simulink model "comparePWM"  (R2023b)
settings: Solver=ode4  StartTime=0.0  StopTime=0.1  FixedStep=Ts  RelTol=1e-3
PreLoadFcn:
  | % Switching
  | fsw = 2e4;
  | Tsw = 1/fsw;
  | Ts = 1e-7;
  | N = 8; % Number of subcycles
  | 
  | DeadTime = 2*Ts; % minimum value
  | 
  | % Default Variants
  | Delay = DelayType.Delay;
  | Inverter = InverterType.Ideal;
  | PWM = PWMType.Def3PhasePWMGen;
  | PWMAccuracy = PWMAccuracyType.Sync;
  | Solver = SolverType.ode4;
  | 
  | % Load Variant Configurations
  | load FastPWMConfigurations.mat;
undefined symbols (not defined in the file or in its folder): TsPWM
libraries: simulink x19, eePwmGenerator x18, nesl_utility x9, ee_lib x7, eePwmGeneratorTwoLevel x3, fl_lib x2, eeGeneralControl x1, eeSinGeneratorThreePhase x1
settings Model: VariantConfigurationObject=FastPWM  Creator=promero  LastModifiedBy=gschrabe
settings SolverCC: ODENIntegrationMethod=ode1be
settings OptimizationCC: ReuseModelBlockBuffer=off
settings ModelReferenceCC: EnableRefExpFcnMdlSchedulingChecks=on

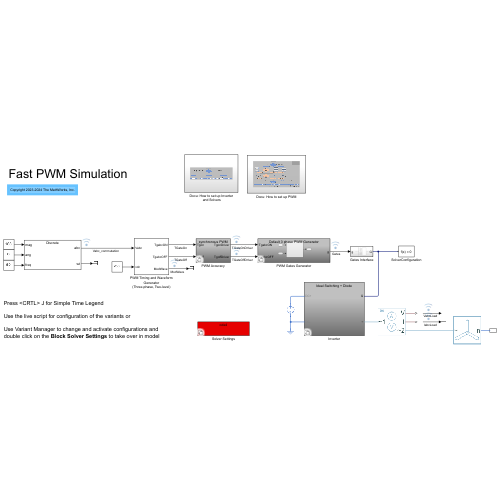
[thumbnail: Simulink's stored preview of the top-level diagram]
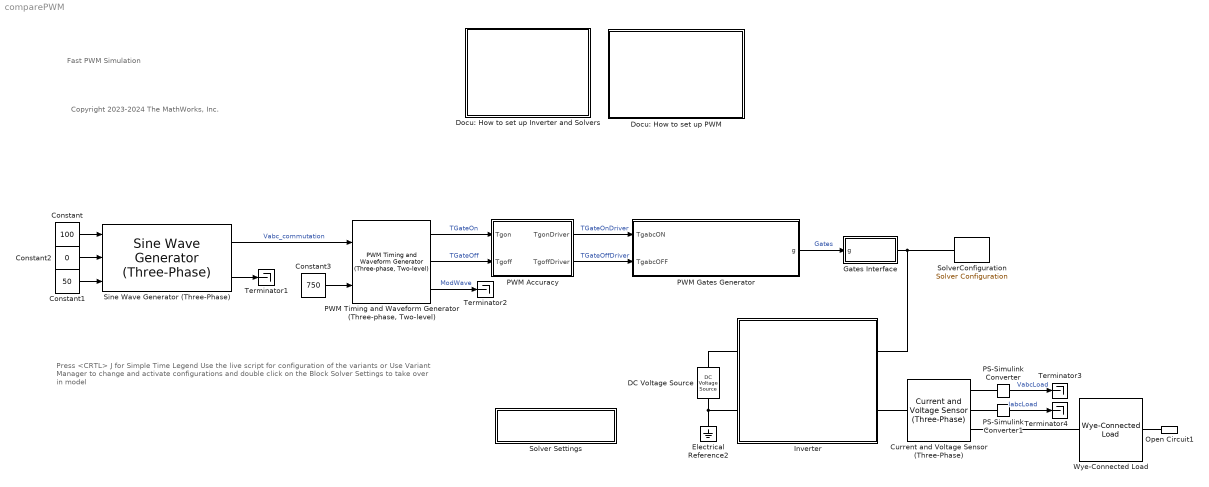
== system comparePWM ==
  note: Copyright 2023-2024 The MathWorks, Inc.
  note: Press <CRTL> J for Simple Time Legend
      |
      | Use the live script for configuration of the variants or
      |
      | Use Variant Manager to change and activate configurations and double click on the Block Solver Settings to take over in model
  note: Fast PWM Simulation
  Constant : Constant  Value=100  SampleTime=Tsw
  Constant1 : Constant  Value=50  SampleTime=Tsw
  Constant2 : Constant  Value=0  SampleTime=Tsw
  Constant3 : Constant  Value=750  SampleTime=Tsw
  Current and Voltage Sensor (Three-Phase) : ee_lib/Sensors & Transducers/Current and Voltage Sensor (Three-Phase)  vMeasurementType=ee.enum.vmeasurement.lg  outputUnit=ee.enum.unit.si  SRated=100e6 A*V  VRated=24e3 V  I_specify=off  I_priority=None  I=[0, 0, 0] A  I_nominal_specify=off  I_nominal_unit=A  I_nominal_value=1  V_specify=off  V_priority=None  V=[0, 0, 0] V  V_nominal_specify=off  V_nominal_unit=V  V_nominal_value=1
      settings: InternalSimscapePortConfiguration="{\"Bottom\":[],\"Left\":[{\"id\":\"N1\",\"label\":\"~1\",\"type\":\"foundation.electrical.three_phase\"}],\"Right\":[{\"id\":\"V_output\",\"label\":\"V\",\"type\":\"output\"},{\"id\":\"I_output\",\"label\":\"I\",\"type\":\"output\"},{\"id\":\"N2\",\"label\":\"~2\",\"type\":\"foundation.electrical.three_phase\"}],\"Top\":[]}"
  DC Voltage Source : ee_lib/Additional Components/SPICE Sources/DC Voltage Source  DC=750 V
  Docu: How to set up Inverter and Solvers : Subsystem
  Docu: How to set up PWM : Subsystem
  Electrical Reference2 : fl_lib/Electrical/Electrical Elements/Electrical Reference
  Gates Interface : Subsystem
  Inverter : Subsystem  Variant=on  VariantControl=Choice
  Open Circuit1 : fl_lib/Electrical/Electrical Elements/Open Circuit  v_specify=off  v_priority=None  v=0 V  v_nominal_specify=off  v_nominal_unit=V  v_nominal_value=1
  PS-Simulink Converter : nesl_utility/PS-Simulink Converter  PhysicalDomain=network_engine_domain  SubClassName=ps_output  LeftPortType=input  RightPortType=output  PseudoPeriodic=off  Frequencies=[]  VectorFormat=inherit  Unit=inherit  AffineConversion=off
  PS-Simulink Converter1 : nesl_utility/PS-Simulink Converter  PhysicalDomain=network_engine_domain  SubClassName=ps_output  LeftPortType=input  RightPortType=output  PseudoPeriodic=off  Frequencies=[]  VectorFormat=inherit  Unit=inherit  AffineConversion=off
  PWM Accuracy : Subsystem  InitFcn=|  Variant=on  VariantControl=Choice
      | if Ts == 0
      |    PWMAccuracy = 0;% ContinuousPWM;
      | else
      |    PWMAccuracy = 1; %DiscretePWM;
      | end
  PWM Gates Generator : Subsystem  Variant=on  VariantControl=Choice
  "PWM Timing and Waveform Generator (Three-phase, Two-level)" : eePwmGeneratorTwoLevel/PWM Timing and Waveform Generator (Three-phase, Two-level)  PWMMode=Continuous PWM (CPWM)  CPWMMode=SVM: space vector modulation  DPWMMode=60 DPWM (-30 degree shift): -30 degree shift from 60 DPWM  fsw=fsw
      settings: SamplingMode=Symmetric
  Sine Wave Generator (Three-Phase) : eeSinGeneratorThreePhase/Sine Wave Generator (Three-Phase)  Ts=Tsw
  Solver Settings : Subsystem  Priority=1  Variant=on  VariantControl=Modelwide Solver Settings
      settings: OpenFcn=open_system(['comparePWM_modified/Solver Settings/',char(Solver)]);
  SolverConfiguration : nesl_utility/Solver Configuration  PhysicalDomain=network_engine_domain  SubClassName=solver  LeftPortType=input  RightPortType=generic  Tones=[]  Harmonics=[]  SimulateNoise=off  Profile=off  UseLocalSampling=off  EnableSwitchedLinearOptims=on  FrequencyDomain=off  UseCCode=off  RelTol=0.001  AbsTol=0.001  MinStep=1e-09  ToWorkspace=off  RevertToSquareIcSolve=off  NumHomotopyIterations=100  PhasorMode=off  PhasorModeNumHarmonics=1  ConsistencySolver=NEWTON_FTOL  IndexReductionMethod=DerivativeReplacement  DoDC=off  ResidualTolerance=1e-09  ConsistencyTolSource=GLOBAL  ConsistencyAbsTol=0.001  ConsistencyRelTol=0.001  ConsistencyTolFactor=0.001  UseLocalSolver=on  LocalSolverChoice=NE_BACKWARD_EULER_ADVANCER  ResolveIndetEquations=on  FunctionEvalNumThread=1  LocalSolverSampleTime=Ts  DoFixedCost=off  MaxNonlinIter=3  MaxModeIter=2  ComputeImpulses=off  ImpulseIterations=2  LinearAlgebra=auto  LinearAlgebraNumThread=0  EquationFormulation=NE_TIME_EF  DelaysMemoryBudget=1024  AutomaticFiltering=on  FilteringTimeConstant=0.001  PartitionStorageMethod=AS_NEEDED  PartitionMemoryBudget=1024  PartitionMethod=ROBUST  MultibodyUseLocalSolver=off  MultibodyLocalSolverChoice=ODE1  MultibodyLocalSolverSampleTime=0.001
  Terminator{1..4} (4 alike) : Terminator
  Wye-Connected Load : ee_lib/Passive/RLC Assemblies/Wye-Connected Load  parameterization=ee.enum.rlc.parameterization.direct  component_structure=ee.enum.rlc.structure.SeriesRL  component_structure_PQ=ee.enum.rlc.structure.SeriesRL  R=1 Ohm  L=1e-3 H  C=1e-6 F  VRated=24e3 V  FRated=60 Hz  P=1e3 W  Qpos=1e2 A*V  Qneg=-1e2 A*V  R_parasitic=0 Ohm  G_parasitic=0 1/Ohm  R_parasitic_PQ=0 Ohm  G_parasitic_PQ=0 1/Ohm  Vmag0=24e3 V  Vang0=0 deg  Freq0=60 Hz  IL_specify=off  IL_priority=High  IL=[0, 0, 0] A  IL_nominal_specify=off  IL_nominal_unit=A  IL_nominal_value=1  VC_specify=off  VC_priority=High  VC=[0, 0, 0] V  VC_nominal_specify=off  VC_nominal_unit=V  VC_nominal_value=1
  wires:
  Constant/1 -> Sine Wave Generator (Three-Phase)/1
  Constant1/1 -> Sine Wave Generator (Three-Phase)/3
  Sine Wave Generator (Three-Phase)/1 -> "PWM Timing and Waveform Generator (Three-phase, Two-level)"/1  "Vabc_commutation"
  Sine Wave Generator (Three-Phase)/2 -> Terminator1/1
  Constant2/1 -> Sine Wave Generator (Three-Phase)/2
  Constant3/1 -> "PWM Timing and Waveform Generator (Three-phase, Two-level)"/2
  "PWM Timing and Waveform Generator (Three-phase, Two-level)"/3 -> Terminator2/1  "ModWave"
  PS-Simulink Converter/1 -> Terminator3/1  "VabcLoad"
  PS-Simulink Converter1/1 -> Terminator4/1  "IabcLoad"
  PWM Gates Generator/1(g) -> Gates Interface/1(g)  "Gates"
  "PWM Timing and Waveform Generator (Three-phase, Two-level)"/1 -> PWM Accuracy/1(Tgon)  "TGateOn"
  "PWM Timing and Waveform Generator (Three-phase, Two-level)"/2 -> PWM Accuracy/2(Tgoff)  "TGateOff"
  PWM Accuracy/1(TgonDriver) -> PWM Gates Generator/1(TgabcON)  "TGateOnDriver"
  PWM Accuracy/2(TgoffDriver) -> PWM Gates Generator/2(TgabcOFF)  "TGateOffDriver"
  connections:
  Wye-Connected Load/LConn1 -- Current and Voltage Sensor (Three-Phase)/RConn3
  PS-Simulink Converter/LConn1 -- Current and Voltage Sensor (Three-Phase)/RConn1
  PS-Simulink Converter1/LConn1 -- Current and Voltage Sensor (Three-Phase)/RConn2
  DC Voltage Source/RConn1 -- Electrical Reference2/LConn1 -- Inverter/RConn2
  Inverter/LConn1 -- SolverConfiguration/RConn1 -- Gates Interface/RConn1
  Inverter/LConn2 -- Current and Voltage Sensor (Three-Phase)/LConn1
  Inverter/RConn1 -- DC Voltage Source/LConn1
  Wye-Connected Load/RConn1 -- Open Circuit1/LConn1

== system comparePWM/Docu: How to set up Inverter and Solvers ==

== system comparePWM/Docu: How to set up PWM ==

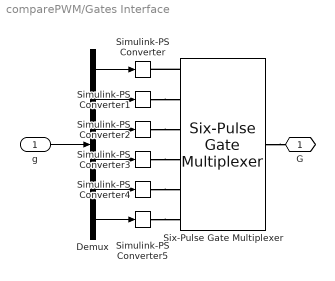
== system comparePWM/Gates Interface ==
  g : Inport
  Demux : Demux  Outputs=6
  Simulink-PS Converter{,1..5} (6 alike) : nesl_utility/Simulink-PS Converter  PhysicalDomain=network_engine_domain  SubClassName=ps_input  LeftPortType=input  RightPortType=output  PseudoPeriodic=off  Frequencies=[]  NoiseDistribution=none  NoiseParameters=[]  Unit=1  AffineConversion=off  FilteringAndDerivatives=provide  SimscapeFilterOrder=1  InputFilterTimeConstant=0.001  UdotUserProvided=0
  Six-Pulse Gate Multiplexer : ee_lib/Semiconductors & Converters/Converters/Six-Pulse Gate Multiplexer  port_option=ee.enum.controlport.ps
  G : PMIOPort  Side=Right
  wires:
  Demux/5 -> Simulink-PS Converter4/1
  Demux/1 -> Simulink-PS Converter/1
  Demux/4 -> Simulink-PS Converter3/1
  Demux/6 -> Simulink-PS Converter5/1
  Demux/2 -> Simulink-PS Converter1/1
  Demux/3 -> Simulink-PS Converter2/1
  g/1 -> Demux/1
  connections:
  Simulink-PS Converter5/RConn1 -- Six-Pulse Gate Multiplexer/LConn6
  Simulink-PS Converter1/RConn1 -- Six-Pulse Gate Multiplexer/LConn2
  Simulink-PS Converter4/RConn1 -- Six-Pulse Gate Multiplexer/LConn5
  Simulink-PS Converter2/RConn1 -- Six-Pulse Gate Multiplexer/LConn3
  Simulink-PS Converter3/RConn1 -- Six-Pulse Gate Multiplexer/LConn4
  Six-Pulse Gate Multiplexer/LConn1 -- Simulink-PS Converter/RConn1
  Six-Pulse Gate Multiplexer/RConn1 -- G/RConn1

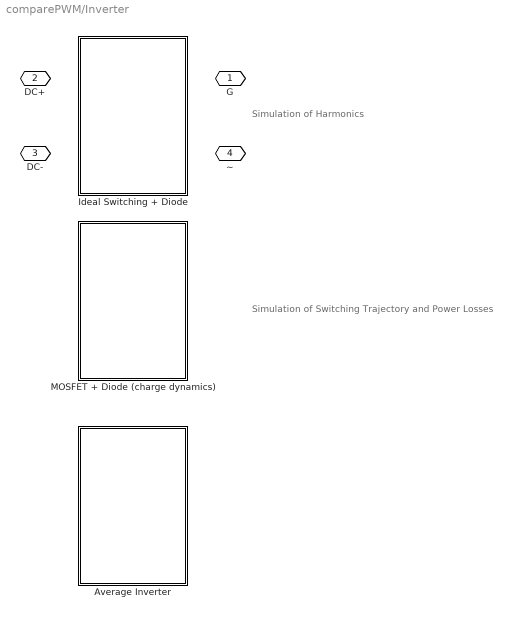
== system comparePWM/Inverter ==
  note: Simulation of Switching Trajectory and Power Losses
  note: Simulation of Harmonics
  Average Inverter : Subsystem  VariantControl=Inverter == InverterType.Average
  Ideal Switching + Diode : Subsystem  VariantControl=Inverter == InverterType.Ideal
  MOSFET + Diode (charge dynamics) : Subsystem  VariantControl=Inverter == InverterType.MOSFET
  G : PMIOPort  Side=Left
  DC+ : PMIOPort  Port=2  Side=Right
  DC- : PMIOPort  Port=3  Side=Right
  ~ : PMIOPort  Port=4  Side=Left

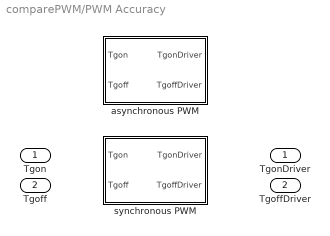
== system comparePWM/PWM Accuracy ==
  Tgon : Inport
  Tgoff : Inport  Port=2
  asynchronous PWM : Subsystem  VariantControl=PWMAccuracy == PWMAccuracyType.Async
  synchronous PWM : Subsystem  VariantControl=PWMAccuracy == PWMAccuracyType.Sync
  TgonDriver : Outport
  TgoffDriver : Outport  Port=2

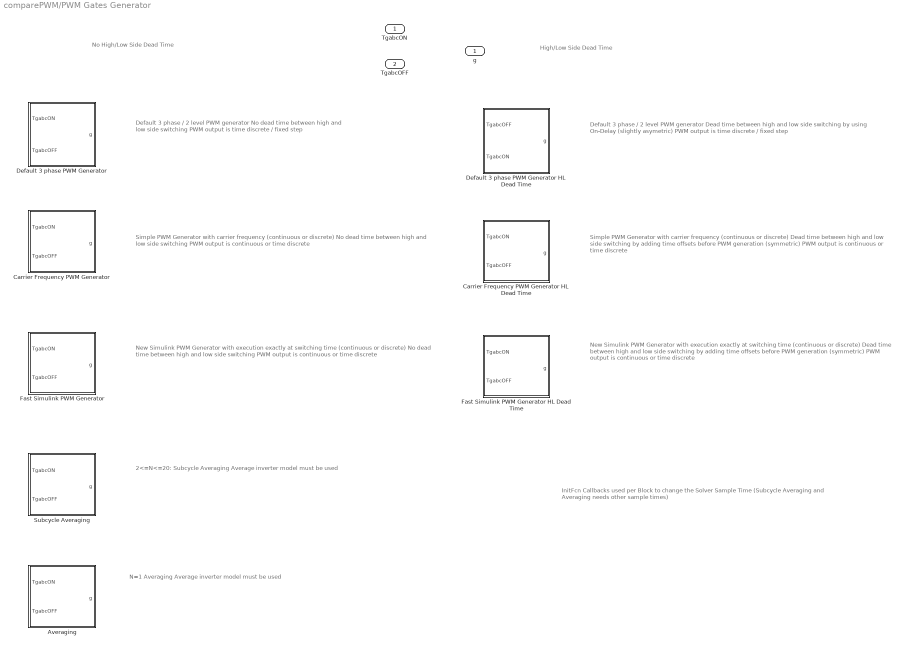
== system comparePWM/PWM Gates Generator ==
  note: InitFcn Callbacks used per Block to change the Solver Sample Time (Subcycle Averaging and Averaging needs other sample times)
  note: No High/Low Side Dead Time
  note: Default 3 phase / 2 level PWM generator
      | No dead time between high and low side switching
      | PWM output is time discrete / fixed step
  note: Default 3 phase / 2 level PWM generator
      | Dead time between high and low side switching by using On-Delay (slightly asymetric)
      | PWM output is time discrete / fixed step
  note: Simple PWM Generator with carrier frequency (continuous or discrete)
      | No dead time between high and low side switching
      | PWM output is continuous or time discrete
  note: Simple PWM Generator with carrier frequency (continuous or discrete)
      | Dead time between high and low side switching by adding time offsets before PWM generation (symmetric)
      | PWM output is continuous or time discrete
  note: New Simulink PWM Generator with execution exactly at switching time (continuous or discrete)
      | No dead time between high and low side switching
      | PWM output is continuous or time discrete
  note: New Simulink PWM Generator with execution exactly at switching time (continuous or discrete)
      | Dead time between high and low side switching by adding time offsets before PWM generation (symmetric)
      | PWM output is continuous or time discrete
  note: High/Low Side Dead Time
  note: 2<=N<=20: Subcycle Averaging
      | Average inverter model must be used
  note: N=1 Averaging
      | Average inverter model must be used
  TgabcON : Inport
  TgabcOFF : Inport  Port=2
  Averaging : Subsystem  InitFcn=|  VariantControl=PWM == PWMType.Averaging  mask{fsw=fsw, N=1}
      | set_param(bdroot,'FixedStep','Tsw');
      | set_param([bdroot,'/SolverConfiguration'],'LocalSolverSampleTime','Tsw');
      mask prompts: fsw "Switching frequency [Hz]"; N "Number of subcycles"
  Carrier Frequency PWM Generator : Subsystem  InitFcn=|  VariantControl=PWM == PWMType.CarrierFreqPWMGen  mask{fsw=fsw, Ts=TsPWM}
      | set_param(bdroot,'FixedStep','Ts');
      | set_param([bdroot,'/SolverConfiguration'],'LocalSolverSampleTime','Ts');
      mask prompts: fsw "Switching frequency [Hz]"; Ts "Sample Time"
  Carrier Frequency PWM Generator HL Dead Time : Subsystem  InitFcn=|  VariantControl=PWM == PWMType.CarrierFreqPWMGenHighLowDeadTime  mask{fsw=fsw, Ts=TsPWM, T_Dead=DeadTime}
      | set_param(bdroot,'FixedStep','Ts');
      | set_param([bdroot,'/SolverConfiguration'],'LocalSolverSampleTime','Ts');
      mask prompts: fsw "Switching frequency [Hz]"; Ts "Sample Time"; T_Dead "PWM dead time high/low side"
  Default 3 phase PWM Generator : Subsystem  InitFcn=|  VariantControl=PWM == PWMType.Def3PhasePWMGen
      | set_param(bdroot,'FixedStep','Ts');
      | set_param([bdroot,'/SolverConfiguration'],'LocalSolverSampleTime','Ts');
  Default 3 phase PWM Generator HL Dead Time : Subsystem  InitFcn=|  VariantControl=PWM == PWMType.Def3PhasePWMGenHighLowDeadTime  mask{fsw=fsw, Ts=Ts, T_Dead=DeadTime}
      | set_param(bdroot,'FixedStep','Ts');
      | set_param([bdroot,'/SolverConfiguration'],'LocalSolverSampleTime','Ts');
      mask prompts: fsw "Switching Frequency"; Ts "Sample Time"; T_Dead "PWM Dead Time High/Low side"
  Fast Simulink PWM Generator : Subsystem  ClipboardFcn=|  VariantControl=PWM == PWMType.FastSimulinkPWMGen  mask{fsw=fsw, Ts=TsPWM}
      | set_param(bdroot,'FixedStep','Ts');
      | set_param([bdroot,'/SolverConfiguration'],'LocalSolverSampleTime','Ts');
      mask prompts: fsw "Switching frequency [Hz]"; Ts "Sample Time"
      mask Callback Ts:
      | if evalin('base',get_param(gcb,'Ts')) == 0
      |         h = find_system(gcb,'LookUnderMasks','on','MatchFilter',@Simulink.match.allVariants,'RunAtFixedTimeIntervals','on');
      |         for i=1:length(h)
      |             set_param(h{i},'RunAtFixedTimeIntervals','off')
      |         end
      |     else
      |         h = find_system(gcb,'LookUnderMasks','on','MatchFilter',@Simulink.match.allVariants,'RunAtFixedTimeIntervals','off');
      |         for i=1:length(h)
      |             set_param(h{i},'RunAtFixedTimeIntervals','on')
      |         end
      |     end
  Fast Simulink PWM Generator HL Dead Time : Subsystem  InitFcn=|  VariantControl=PWM == PWMType.FastSimulinkPWMGenHighLowDeadTime  mask{fsw=fsw, T_Dead=DeadTime, Ts=TsPWM}
      | set_param(bdroot,'FixedStep','Ts');
      | set_param([bdroot,'/SolverConfiguration'],'LocalSolverSampleTime','Ts');
      mask prompts: fsw "Switching frequency [Hz]"; T_Dead "PWM dead time high/low side"; Ts "Sample Time"
      mask Callback Ts:
      | if evalin('base',get_param(gcb,'Ts')) == 0
      |         h = find_system(gcb,'LookUnderMasks','on','MatchFilter',@Simulink.match.allVariants,'RunAtFixedTimeIntervals','on');
      |         for i=1:length(h)
      |             set_param(h{i},'RunAtFixedTimeIntervals','off')
      |         end
      |     else
      |         h = find_system(gcb,'LookUnderMasks','on','MatchFilter',@Simulink.match.allVariants,'RunAtFixedTimeIntervals','off');
      |         for i=1:length(h)
      |             set_param(h{i},'RunAtFixedTimeIntervals','on')
      |         end
      |     end
  Subcycle Averaging : Subsystem  InitFcn=|  VariantControl=PWM == PWMType.SubcycleAvg  mask{fsw=fsw, N=N}
      | set_param(bdroot,'FixedStep','Tsw/N');
      | set_param([bdroot,'/SolverConfiguration'],'LocalSolverSampleTime','Tsw/N');
      mask prompts: fsw "Switching frequency [Hz]"; N "Number of subcycles"
  g : Outport

== system comparePWM/Solver Settings ==
  note: The global solver is changed depending on selected variant
      | This happens with predefined configuration sets
      | Also the Simscape lcoal solver setting is changed here.
  ode23t : Subsystem  VariantControl=Solver == SolverType.ode23t
      settings: OpenFcn=|
      | mdl = bdroot;
      | setActiveConfigSet(mdl,'ode23t');
      | set_param([mdl,'/SolverConfiguration'],'UseLocalSolver','off');
      | TsPWM = 0;
  ode4 : Subsystem  VariantControl=Solver == SolverType.ode4
      settings: OpenFcn=|
      | mdl = bdroot;
      | setActiveConfigSet(mdl,'ode4');
      | set_param([mdl,'/SolverConfiguration'],'UseLocalSolver','on');
      |         set_param([mdl,'/SolverConfiguration'],'LocalSolverChoice','NE_BACKWARD_EULER_ADVANCER');
      |         set_param([mdl,'/SolverConfiguration'],'LocalSolverSampleTime','Ts');
      | TsPWM = Ts;
  odeN : Subsystem  VariantControl=Solver == SolverType.odeN
      settings: OpenFcn=|
      | mdl = bdroot;
      | setActiveConfigSet(mdl,'odeN');
      | set_param([mdl,'/SolverConfiguration'],'UseLocalSolver','off');
      | TsPWM = 0;

== system comparePWM/Inverter/Average Inverter ==
  Converter (Three-Phase) : ee_lib/Semiconductors & Converters/Converters/Converter (Three-Phase)  port_option=ee.enum.threePhasePort.composite  device_type=ee.enum.converters.switchingdevice.averaged  K=0  Vf=0.8 V  Ron=0.001 Ohm  Rds=0.001 Ohm  Goff=1e-6 1/Ohm  Vgt=1 V  Vgt_off=-1 V  Ih=1 A  Vth=0.5 V  diode_param=ee.enum.converters.protectiondiode.chargedynamics  diode_Vf=0.8 V  diode_Ron=0.001 Ohm  diode_Goff=1e-5 1/Ohm  diode_C=50 nF  diode_iRM=-235 A  diode_iF=300 A  diode_idot=-50 A/us  diode_trr_param=ee.enum.converters.diodetrr.trr_factor  diode_trr_factor=3  diode_trr=15 us  diode_Qrr=1500 s*uA  snubber_type=ee.enum.converters.snubber.exclude  Cs=1e-7 F  Rs=0.1 Ohm
  G : PMIOPort  Side=Left
  DC+ : PMIOPort  Port=2  Side=Right
  DC- : PMIOPort  Port=3  Side=Right
  ~ : PMIOPort  Port=4  Side=Left
  connections:
  Converter (Three-Phase)/RConn1 -- DC+/RConn1
  Converter (Three-Phase)/RConn2 -- DC-/RConn1
  G/RConn1 -- Converter (Three-Phase)/LConn1
  ~/RConn1 -- Converter (Three-Phase)/LConn2

== system comparePWM/Inverter/Ideal Switching + Diode ==
  Converter (Three-Phase) : ee_lib/Semiconductors & Converters/Converters/Converter (Three-Phase)  port_option=ee.enum.threePhasePort.composite  device_type=ee.enum.converters.switchingdevice.ideal  K=0  Vf=0.8 V  Ron=0.001 Ohm  Rds=0.001 Ohm  Goff=1e-6 1/Ohm  Vgt=1 V  Vgt_off=-1 V  Ih=1 A  Vth=0.5 V  diode_param=ee.enum.converters.protectiondiode.nodynamics  diode_Vf=0.8 V  diode_Ron=0.001 Ohm  diode_Goff=1e-5 1/Ohm  diode_C=50 nF  diode_iRM=-235 A  diode_iF=300 A  diode_idot=-50 A/us  diode_trr_param=ee.enum.converters.diodetrr.trr_factor  diode_trr_factor=3  diode_trr=15 us  diode_Qrr=1500 s*uA  snubber_type=ee.enum.converters.snubber.exclude  Cs=1e-7 F  Rs=0.1 Ohm
  G : PMIOPort  Side=Left
  DC+ : PMIOPort  Port=2  Side=Right
  DC- : PMIOPort  Port=3  Side=Right
  ~ : PMIOPort  Port=4  Side=Left
  connections:
  Converter (Three-Phase)/RConn1 -- DC+/RConn1
  Converter (Three-Phase)/RConn2 -- DC-/RConn1
  G/RConn1 -- Converter (Three-Phase)/LConn1
  ~/RConn1 -- Converter (Three-Phase)/LConn2

== system comparePWM/Inverter/MOSFET + Diode (charge dynamics) ==
  Converter (Three-Phase) : ee_lib/Semiconductors & Converters/Converters/Converter (Three-Phase)  port_option=ee.enum.threePhasePort.composite  device_type=ee.enum.converters.switchingdevice.mosfet  K=0  Vf=0.8 V  Ron=0.001 Ohm  Rds=0.001 Ohm  Goff=1e-6 1/Ohm  Vgt=1 V  Vgt_off=-1 V  Ih=1 A  Vth=0.5 V  diode_param=ee.enum.converters.protectiondiode.chargedynamics  diode_Vf=0.8 V  diode_Ron=0.001 Ohm  diode_Goff=1e-5 1/Ohm  diode_C=50 nF  diode_iRM=-235 A  diode_iF=300 A  diode_idot=-50 A/us  diode_trr_param=ee.enum.converters.diodetrr.trr_factor  diode_trr_factor=3  diode_trr=15 us  diode_Qrr=1500 s*uA  snubber_type=ee.enum.converters.snubber.exclude  Cs=1e-7 F  Rs=0.1 Ohm
  G : PMIOPort  Side=Left
  DC+ : PMIOPort  Port=2  Side=Right
  DC- : PMIOPort  Port=3  Side=Right
  ~ : PMIOPort  Port=4  Side=Left
  connections:
  ~/RConn1 -- Converter (Three-Phase)/LConn2
  G/RConn1 -- Converter (Three-Phase)/LConn1
  Converter (Three-Phase)/RConn2 -- DC-/RConn1
  Converter (Three-Phase)/RConn1 -- DC+/RConn1

== system comparePWM/PWM Accuracy/asynchronous PWM ==
  note: Take exact PWM switching times
  Tgon : Inport
  Tgoff : Inport  Port=2
  TgonDriver : Outport
  TgoffDriver : Outport  Port=2
  wires:
  Tgoff/1 -> TgoffDriver/1
  Tgon/1 -> TgonDriver/1

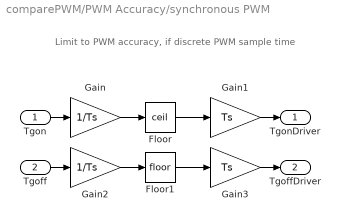
== system comparePWM/PWM Accuracy/synchronous PWM ==
  note: Limit to PWM accuracy, if discrete PWM sample time
  Tgon : Inport
  Tgoff : Inport  Port=2
  Floor : Rounding  Operator=ceil
  Floor1 : Rounding
  Gain : Gain  Gain=1/Ts
  Gain1 : Gain  Gain=Ts
  Gain2 : Gain  Gain=1/Ts
  Gain3 : Gain  Gain=Ts
  TgonDriver : Outport
  TgoffDriver : Outport  Port=2
  wires:
  Floor1/1 -> Gain3/1
  Gain1/1 -> TgonDriver/1
  Gain/1 -> Floor/1
  Gain2/1 -> Floor1/1
  Floor/1 -> Gain1/1
  Tgoff/1 -> Gain2/1
  Gain3/1 -> TgoffDriver/1
  Tgon/1 -> Gain/1

== system comparePWM/PWM Gates Generator/Averaging ==
  TgabcON : Inport
  TgabcOFF : Inport  Port=2
  Averaging : Subsystem  mask{fsw=fsw, N=N}
      mask prompts: fsw "Switching Frequency"; N "Number of Subcycles (2<=N<=20)"
  Delay : Subsystem  Variant=on  VariantControl=Choice
  g : Outport
  wires:
  Averaging/1(DC) -> g/1
  TgabcON/1 -> Delay/1(On)  "DutyCycleON"
  TgabcOFF/1 -> Delay/2(Off)  "DutyCycleOFF"
  Delay/1(On_Dly) -> Averaging/1(TgabcON)
  Delay/2(Off_Dly) -> Averaging/2(TgabcOFF)

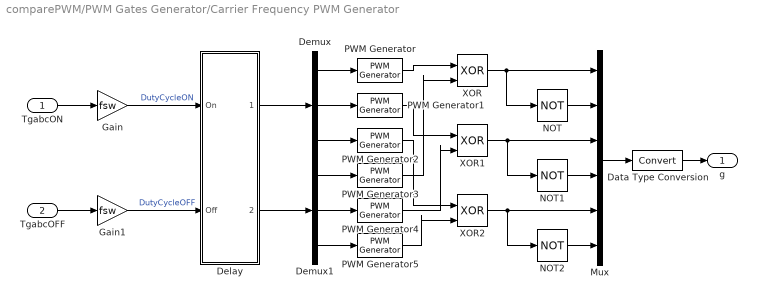
== system comparePWM/PWM Gates Generator/Carrier Frequency PWM Generator ==
  TgabcON : Inport
  TgabcOFF : Inport  Port=2
  Data Type Conversion : DataTypeConversion  SaturateOnIntegerOverflow=off  RndMeth=Floor
  Delay : Subsystem  Variant=on  VariantControl=Choice
  Demux : Demux  Outputs=3
  Demux1 : Demux  Outputs=3
  Gain : Gain  Gain=fsw
  Gain1 : Gain  Gain=fsw
  Mux : Mux  Inputs=6
  NOT : Logic  Operator=NOT  IconShape=distinctive  AllPortsSameDT=off  OutDataTypeStr=boolean
  NOT1 : Logic  Operator=NOT  IconShape=distinctive  AllPortsSameDT=off  OutDataTypeStr=boolean
  NOT2 : Logic  Operator=NOT  IconShape=distinctive  AllPortsSameDT=off  OutDataTypeStr=boolean
  PWM Generator{,1..5} (6 alike) : eePwmGenerator/PWM Generator  CarrCount=Up  Tper=1/fsw  Tdelay=0  Ts=Ts
  XOR : Logic  Operator=XOR  IconShape=distinctive  AllPortsSameDT=off  OutDataTypeStr=boolean
  XOR1 : Logic  Operator=XOR  IconShape=distinctive  AllPortsSameDT=off  OutDataTypeStr=boolean
  XOR2 : Logic  Operator=XOR  IconShape=distinctive  AllPortsSameDT=off  OutDataTypeStr=boolean
  g : Outport
  wires:
  NOT2/1 -> Mux/6
  NOT1/1 -> Mux/4
  NOT/1 -> Mux/2
  XOR1/1 -> Mux/3, NOT1/1
  XOR2/1 -> Mux/5, NOT2/1
  XOR/1 -> Mux/1, NOT/1
  PWM Generator5/1 -> XOR2/2
  PWM Generator2/1 -> XOR2/1
  PWM Generator4/1 -> XOR1/2
  PWM Generator1/1 -> XOR1/1
  PWM Generator3/1 -> XOR/2
  PWM Generator/1 -> XOR/1
  TgabcOFF/1 -> Gain1/1
  Mux/1 -> Data Type Conversion/1
  TgabcON/1 -> Gain/1
  Data Type Conversion/1 -> g/1
  Demux/1 -> PWM Generator/1
  Demux/2 -> PWM Generator1/1
  Demux/3 -> PWM Generator2/1
  Demux1/1 -> PWM Generator3/1
  Demux1/2 -> PWM Generator4/1
  Demux1/3 -> PWM Generator5/1
  Gain/1 -> Delay/1(On)  "DutyCycleON"
  Gain1/1 -> Delay/2(Off)  "DutyCycleOFF"
  Delay/1(On_Dly) -> Demux/1
  Delay/2(Off_Dly) -> Demux1/1

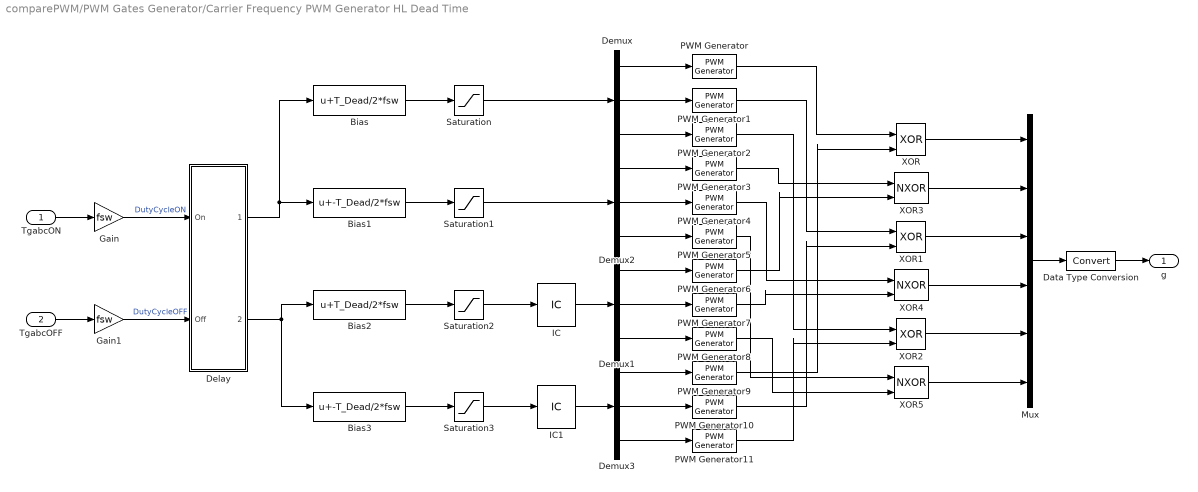
== system comparePWM/PWM Gates Generator/Carrier Frequency PWM Generator HL Dead Time ==
  TgabcON : Inport
  TgabcOFF : Inport  Port=2
  Bias : Bias  Bias=T_Dead/2*fsw  SaturateOnIntegerOverflow=off
  Bias1 : Bias  Bias=-T_Dead/2*fsw  SaturateOnIntegerOverflow=off
  Bias2 : Bias  Bias=T_Dead/2*fsw  SaturateOnIntegerOverflow=off
  Bias3 : Bias  Bias=-T_Dead/2*fsw  SaturateOnIntegerOverflow=off
  Data Type Conversion : DataTypeConversion  SaturateOnIntegerOverflow=off  RndMeth=Floor
  Delay : Subsystem  Variant=on  VariantControl=Choice
  Demux{,1..3} (4 alike) : Demux  Outputs=3
  Gain : Gain  Gain=fsw
  Gain1 : Gain  Gain=fsw
  IC : InitialCondition  Value=[0 0 0]
  IC1 : InitialCondition  Value=[0 0 0]
  Mux : Mux  Inputs=6
  PWM Generator{,1..11} (12 alike) : eePwmGenerator/PWM Generator  CarrCount=Up  Tper=1/fsw  Tdelay=0  Ts=Ts
  Saturation : Saturate  UpperLimit=1/2  LowerLimit=0
  Saturation1 : Saturate  UpperLimit=1/2  LowerLimit=0
  Saturation2 : Saturate  UpperLimit=1  LowerLimit=1/2
  Saturation3 : Saturate  UpperLimit=1  LowerLimit=1/2
  XOR : Logic  Operator=XOR  IconShape=distinctive  AllPortsSameDT=off  OutDataTypeStr=boolean
  XOR1 : Logic  Operator=XOR  IconShape=distinctive  AllPortsSameDT=off  OutDataTypeStr=boolean
  XOR2 : Logic  Operator=XOR  IconShape=distinctive  AllPortsSameDT=off  OutDataTypeStr=boolean
  XOR3 : Logic  Operator=NXOR  IconShape=distinctive  AllPortsSameDT=off  OutDataTypeStr=boolean
  XOR4 : Logic  Operator=NXOR  IconShape=distinctive  AllPortsSameDT=off  OutDataTypeStr=boolean
  XOR5 : Logic  Operator=NXOR  IconShape=distinctive  AllPortsSameDT=off  OutDataTypeStr=boolean
  g : Outport
  wires:
  Delay/1(On_Dly) -> Bias/1, Bias1/1
  Saturation3/1 -> IC1/1
  Saturation2/1 -> IC/1
  Saturation1/1 -> Demux2/1
  Saturation/1 -> Demux/1
  PWM Generator8/1 -> XOR5/2
  PWM Generator5/1 -> XOR5/1
  PWM Generator7/1 -> XOR4/2
  PWM Generator4/1 -> XOR4/1
  PWM Generator3/1 -> XOR3/1
  PWM Generator11/1 -> XOR2/2
  PWM Generator2/1 -> XOR2/1
  PWM Generator10/1 -> XOR1/2
  PWM Generator1/1 -> XOR1/1
  PWM Generator/1 -> XOR/1
  PWM Generator9/1 -> XOR/2
  PWM Generator6/1 -> XOR3/2
  Bias3/1 -> Saturation3/1
  Demux3/3 -> PWM Generator11/1
  Demux3/2 -> PWM Generator10/1
  Demux3/1 -> PWM Generator9/1
  Demux1/3 -> PWM Generator8/1
  Demux1/2 -> PWM Generator7/1
  Demux1/1 -> PWM Generator6/1
  Bias1/1 -> Saturation1/1
  Demux2/3 -> PWM Generator5/1
  Demux2/2 -> PWM Generator4/1
  Demux2/1 -> PWM Generator3/1
  Demux/3 -> PWM Generator2/1
  Demux/2 -> PWM Generator1/1
  Demux/1 -> PWM Generator/1
  Bias2/1 -> Saturation2/1
  Bias/1 -> Saturation/1
  Mux/1 -> Data Type Conversion/1
  TgabcOFF/1 -> Gain1/1
  TgabcON/1 -> Gain/1
  XOR/1 -> Mux/1
  XOR2/1 -> Mux/5
  XOR1/1 -> Mux/3
  XOR3/1 -> Mux/2
  XOR4/1 -> Mux/4
  XOR5/1 -> Mux/6
  Data Type Conversion/1 -> g/1
  Gain/1 -> Delay/1(On)  "DutyCycleON"
  Gain1/1 -> Delay/2(Off)  "DutyCycleOFF"
  Delay/2(Off_Dly) -> Bias2/1, Bias3/1
  IC/1 -> Demux1/1
  IC1/1 -> Demux3/1

== system comparePWM/PWM Gates Generator/Default 3 phase PWM Generator ==
  TgabcON : Inport
  TgabcOFF : Inport  Port=2
  Default 3 phase PWM Generator : eePwmGeneratorTwoLevel/PWM Gate Signal Generator (Three-phase, Two-level)  VariantControl=PWM == PWMType.Def3PhasePWMGen  fsw=fsw  Ts=Ts
      settings: SamplingMode=Symmetric
  g : Outport
  wires:
  TgabcON/1 -> Default 3 phase PWM Generator/1
  TgabcOFF/1 -> Default 3 phase PWM Generator/2
  Default 3 phase PWM Generator/1 -> g/1

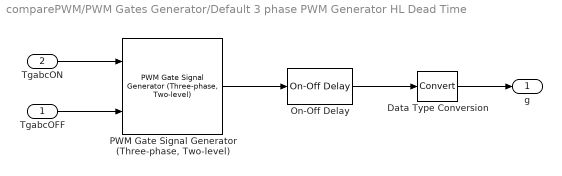
== system comparePWM/PWM Gates Generator/Default 3 phase PWM Generator HL Dead Time ==
  TgabcOFF : Inport
  TgabcON : Inport  Port=2
  Data Type Conversion : DataTypeConversion  SaturateOnIntegerOverflow=off  RndMeth=Floor
  On-Off Delay : eeGeneralControl/On-Off Delay  LabelModeActiveChoice=Discrete  Td_on=T_Dead  Td_off=0  IC=0  Ts=Ts
      settings: LibrarySourceBlock=ee_sl_lib/General Control/On-Off Delay
  "PWM Gate Signal Generator (Three-phase, Two-level)" : eePwmGeneratorTwoLevel/PWM Gate Signal Generator (Three-phase, Two-level)  fsw=fsw  Ts=Ts
      settings: SamplingMode=Symmetric
  g : Outport
  wires:
  TgabcON/1 -> "PWM Gate Signal Generator (Three-phase, Two-level)"/1
  TgabcOFF/1 -> "PWM Gate Signal Generator (Three-phase, Two-level)"/2
  "PWM Gate Signal Generator (Three-phase, Two-level)"/1 -> On-Off Delay/1
  On-Off Delay/1 -> Data Type Conversion/1
  Data Type Conversion/1 -> g/1

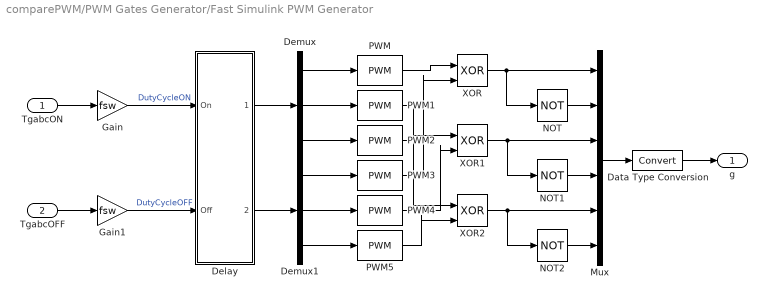
== system comparePWM/PWM Gates Generator/Fast Simulink PWM Generator ==
  TgabcON : Inport
  TgabcOFF : Inport  Port=2
  Data Type Conversion : DataTypeConversion  SaturateOnIntegerOverflow=off  RndMeth=Floor
  Delay : Subsystem  Variant=on  VariantControl=Choice
  Demux : Demux  Outputs=3
  Demux1 : Demux  Outputs=3
  Gain : Gain  Gain=fsw
  Gain1 : Gain  Gain=fsw
  Mux : Mux  Inputs=6
  NOT : Logic  Operator=NOT  IconShape=distinctive  AllPortsSameDT=off  OutDataTypeStr=boolean
  NOT1 : Logic  Operator=NOT  IconShape=distinctive  AllPortsSameDT=off  OutDataTypeStr=boolean
  NOT2 : Logic  Operator=NOT  IconShape=distinctive  AllPortsSameDT=off  OutDataTypeStr=boolean
  PWM{,1..5} (6 alike) : simulink/Discontinuities/PWM  DisableCoverage=on  Period=1/fsw  InitialDelay=0  DisallowZeroDutyCycle=off  RunAtFixedTimeIntervals=off  SampleTime=Ts
  XOR : Logic  Operator=XOR  IconShape=distinctive  AllPortsSameDT=off  OutDataTypeStr=boolean
  XOR1 : Logic  Operator=XOR  IconShape=distinctive  AllPortsSameDT=off  OutDataTypeStr=boolean
  XOR2 : Logic  Operator=XOR  IconShape=distinctive  AllPortsSameDT=off  OutDataTypeStr=boolean
  g : Outport
  wires:
  Mux/1 -> Data Type Conversion/1
  Demux1/3 -> PWM5/1
  Demux1/2 -> PWM4/1
  Demux1/1 -> PWM3/1
  Demux/3 -> PWM2/1
  Demux/2 -> PWM1/1
  Demux/1 -> PWM/1
  TgabcOFF/1 -> Gain1/1
  TgabcON/1 -> Gain/1
  PWM/1 -> XOR/1
  PWM3/1 -> XOR/2
  PWM1/1 -> XOR1/1
  PWM4/1 -> XOR1/2
  PWM2/1 -> XOR2/1
  PWM5/1 -> XOR2/2
  XOR/1 -> NOT/1, Mux/1
  XOR2/1 -> NOT2/1, Mux/5
  XOR1/1 -> NOT1/1, Mux/3
  NOT/1 -> Mux/2
  NOT1/1 -> Mux/4
  NOT2/1 -> Mux/6
  Data Type Conversion/1 -> g/1
  Gain/1 -> Delay/1(On)  "DutyCycleON"
  Gain1/1 -> Delay/2(Off)  "DutyCycleOFF"
  Delay/1(On_Dly) -> Demux/1
  Delay/2(Off_Dly) -> Demux1/1

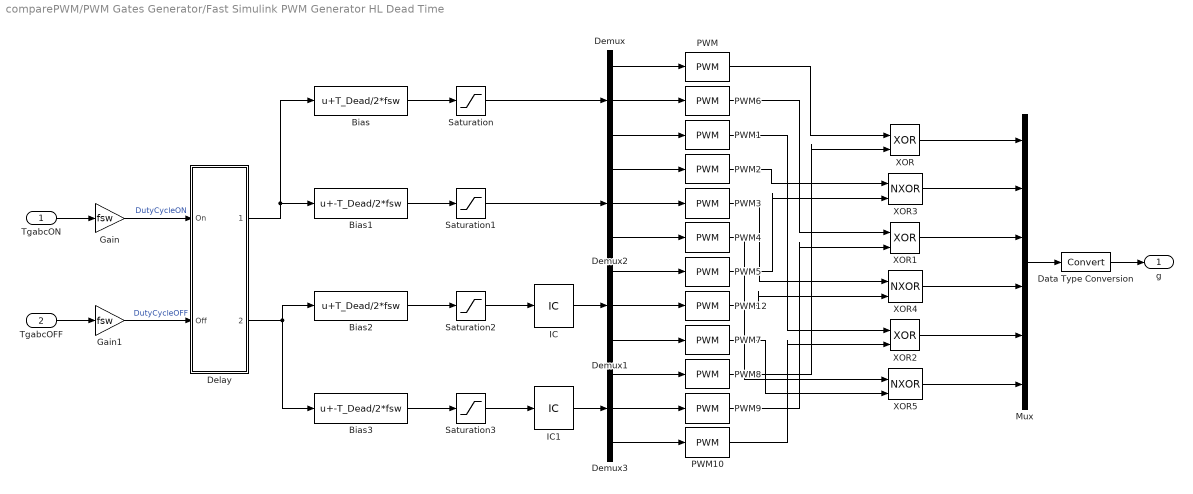
== system comparePWM/PWM Gates Generator/Fast Simulink PWM Generator HL Dead Time ==
  TgabcON : Inport
  TgabcOFF : Inport  Port=2
  Bias : Bias  Bias=T_Dead/2*fsw  SaturateOnIntegerOverflow=off
  Bias1 : Bias  Bias=-T_Dead/2*fsw  SaturateOnIntegerOverflow=off
  Bias2 : Bias  Bias=T_Dead/2*fsw  SaturateOnIntegerOverflow=off
  Bias3 : Bias  Bias=-T_Dead/2*fsw  SaturateOnIntegerOverflow=off
  Data Type Conversion : DataTypeConversion  SaturateOnIntegerOverflow=off  RndMeth=Floor
  Delay : Subsystem  Variant=on  VariantControl=Choice
  Demux{,1..3} (4 alike) : Demux  Outputs=3
  Gain : Gain  Gain=fsw
  Gain1 : Gain  Gain=fsw
  IC : InitialCondition  Value=[0 0 0]
  IC1 : InitialCondition  Value=[0 0 0]
  Mux : Mux  Inputs=6
  PWM{,1..10,12} (12 alike) : simulink/Discontinuities/PWM  DisableCoverage=on  Period=1/fsw  InitialDelay=0  DisallowZeroDutyCycle=off  RunAtFixedTimeIntervals=on  SampleTime=Ts
  Saturation : Saturate  UpperLimit=1/2  LowerLimit=0
  Saturation1 : Saturate  UpperLimit=1/2  LowerLimit=0
  Saturation2 : Saturate  UpperLimit=1  LowerLimit=1/2
  Saturation3 : Saturate  UpperLimit=1  LowerLimit=1/2
  XOR : Logic  Operator=XOR  IconShape=distinctive  AllPortsSameDT=off  OutDataTypeStr=boolean
  XOR1 : Logic  Operator=XOR  IconShape=distinctive  AllPortsSameDT=off  OutDataTypeStr=boolean
  XOR2 : Logic  Operator=XOR  IconShape=distinctive  AllPortsSameDT=off  OutDataTypeStr=boolean
  XOR3 : Logic  Operator=NXOR  IconShape=distinctive  AllPortsSameDT=off  OutDataTypeStr=boolean
  XOR4 : Logic  Operator=NXOR  IconShape=distinctive  AllPortsSameDT=off  OutDataTypeStr=boolean
  XOR5 : Logic  Operator=NXOR  IconShape=distinctive  AllPortsSameDT=off  OutDataTypeStr=boolean
  g : Outport
  wires:
  Delay/2(Off_Dly) -> Bias3/1, Bias2/1
  Gain1/1 -> Delay/2(Off)  "DutyCycleOFF"
  Gain/1 -> Delay/1(On)  "DutyCycleON"
  Data Type Conversion/1 -> g/1
  XOR5/1 -> Mux/6
  XOR4/1 -> Mux/4
  XOR3/1 -> Mux/2
  XOR1/1 -> Mux/3
  XOR2/1 -> Mux/5
  XOR/1 -> Mux/1
  TgabcON/1 -> Gain/1
  TgabcOFF/1 -> Gain1/1
  Mux/1 -> Data Type Conversion/1
  Bias/1 -> Saturation/1
  Bias2/1 -> Saturation2/1
  Demux/1 -> PWM/1
  Demux/2 -> PWM6/1
  Demux/3 -> PWM1/1
  Demux2/1 -> PWM2/1
  Demux2/2 -> PWM3/1
  Demux2/3 -> PWM4/1
  Bias1/1 -> Saturation1/1
  Demux1/1 -> PWM5/1
  Demux1/2 -> PWM12/1
  Demux1/3 -> PWM7/1
  Demux3/1 -> PWM8/1
  Demux3/2 -> PWM9/1
  Demux3/3 -> PWM10/1
  Bias3/1 -> Saturation3/1
  PWM5/1 -> XOR3/2
  PWM8/1 -> XOR/2
  PWM/1 -> XOR/1
  PWM6/1 -> XOR1/1
  PWM9/1 -> XOR1/2
  PWM1/1 -> XOR2/1
  PWM10/1 -> XOR2/2
  PWM2/1 -> XOR3/1
  PWM3/1 -> XOR4/1
  PWM12/1 -> XOR4/2
  PWM4/1 -> XOR5/1
  PWM7/1 -> XOR5/2
  Saturation/1 -> Demux/1
  Saturation1/1 -> Demux2/1
  Saturation2/1 -> IC/1
  Saturation3/1 -> IC1/1
  Delay/1(On_Dly) -> Bias1/1, Bias/1
  IC1/1 -> Demux3/1
  IC/1 -> Demux1/1

== system comparePWM/PWM Gates Generator/Subcycle Averaging ==
  TgabcON : Inport
  TgabcOFF : Inport  Port=2
  Delay : Subsystem  Variant=on  VariantControl=Choice
  SubcycleAveraging : Subsystem  mask{fsw=fsw, N=N}
      mask prompts: fsw "Switching Frequency"; N "Number of Subcycles (2<=N<=20)"
  g : Outport
  wires:
  Delay/2(Off_Dly) -> SubcycleAveraging/2(TgabcOFF)
  Delay/1(On_Dly) -> SubcycleAveraging/1(TgabcON)
  TgabcOFF/1 -> Delay/2(Off)  "DutyCycleOFF"
  TgabcON/1 -> Delay/1(On)  "DutyCycleON"
  SubcycleAveraging/1(DC) -> g/1

== system comparePWM/Solver Settings/ode23t ==

== system comparePWM/Solver Settings/ode4 ==

== system comparePWM/Solver Settings/odeN ==

== system comparePWM/PWM Gates Generator/Averaging/Averaging ==
  TgabcON : Inport
  TgabcOFF : Inport  Port=2
  Calculate Average Duty Cycles : MATLAB Function  TreatAsAtomicUnit=on
  DC : Outport
  wires:
  Calculate Average Duty Cycles/1(DC) -> DC/1
  TgabcON/1 -> Calculate Average Duty Cycles/1(TgabcON)
  TgabcOFF/1 -> Calculate Average Duty Cycles/2(TgabcOFF)

== system comparePWM/PWM Gates Generator/Averaging/Delay ==
  On : Inport
  Off : Inport  Port=2
  Delay : Subsystem  VariantControl=Delay == DelayType.Delay
  NoDelay : Subsystem  VariantControl=Delay == DelayType.NoDelay
  On_Dly : Outport
  Off_Dly : Outport  Port=2

== system comparePWM/PWM Gates Generator/Carrier Frequency PWM Generator/Delay ==
  On : Inport
  Off : Inport  Port=2
  Delay : Subsystem  VariantControl=Delay == DelayType.Delay
  NoDelay : Subsystem  VariantControl=Delay == DelayType.NoDelay
  On_Dly : Outport
  Off_Dly : Outport  Port=2

== system comparePWM/PWM Gates Generator/Carrier Frequency PWM Generator HL Dead Time/Delay ==
  On : Inport
  Off : Inport  Port=2
  Delay : Subsystem  VariantControl=Delay == DelayType.Delay
  NoDelay : Subsystem  VariantControl=Delay == DelayType.NoDelay
  On_Dly : Outport
  Off_Dly : Outport  Port=2

== system comparePWM/PWM Gates Generator/Fast Simulink PWM Generator/Delay ==
  On : Inport
  Off : Inport  Port=2
  Delay : Subsystem  VariantControl=Delay == DelayType.Delay
  NoDelay : Subsystem  VariantControl=Delay == DelayType.NoDelay
  On_Dly : Outport
  Off_Dly : Outport  Port=2

== system comparePWM/PWM Gates Generator/Fast Simulink PWM Generator HL Dead Time/Delay ==
  On : Inport
  Off : Inport  Port=2
  Delay : Subsystem  VariantControl=Delay == DelayType.Delay
  NoDelay : Subsystem  VariantControl=Delay == DelayType.NoDelay
  On_Dly : Outport
  Off_Dly : Outport  Port=2

== system comparePWM/PWM Gates Generator/Subcycle Averaging/Delay ==
  On : Inport
  Off : Inport  Port=2
  Delay : Subsystem  VariantControl=Delay == DelayType.Delay
  NoDelay : Subsystem  VariantControl=Delay == DelayType.NoDelay
  On_Dly : Outport
  Off_Dly : Outport  Port=2

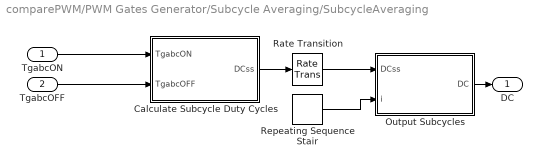
== system comparePWM/PWM Gates Generator/Subcycle Averaging/SubcycleAveraging ==
  TgabcON : Inport
  TgabcOFF : Inport  Port=2
  Calculate Subcycle Duty Cycles : MATLAB Function  TreatAsAtomicUnit=on
  Output Subcycles : MATLAB Function  TreatAsAtomicUnit=on
  Rate Transition : RateTransition  Integrity=off  Deterministic=off  InitialCondition=zeros(N,3)  OutPortSampleTime=1/fsw/N
  Repeating Sequence Stair : simulink/Sources/Repeating Sequence Stair  OutValues=1:N  tsamp=1/fsw/N  OutMin=[]  OutMax=[]  OutDataTypeStr=double  OutputDataTypeScalingMode=double  OutDataType=fixdt(0,8)  ConRadixGroup=Best Precision: Vector-wise  OutScaling=2^-12
  DC : Outport
  wires:
  Calculate Subcycle Duty Cycles/1(DCss) -> Rate Transition/1
  Rate Transition/1 -> Output Subcycles/1(DCss)
  Repeating Sequence Stair/1 -> Output Subcycles/2(i)
  TgabcON/1 -> Calculate Subcycle Duty Cycles/1(TgabcON)
  TgabcOFF/1 -> Calculate Subcycle Duty Cycles/2(TgabcOFF)
  Output Subcycles/1(DC) -> DC/1

== system comparePWM/PWM Gates Generator/Averaging/Delay/Delay ==
  On : Inport
  Off : Inport  Port=2
  Unit Delay : UnitDelay  SampleTime=1/fsw  HasFrameUpgradeWarning=on
  Unit Delay1 : UnitDelay  SampleTime=1/fsw  HasFrameUpgradeWarning=on
  On_Dly : Outport
  Off_Dly : Outport  Port=2
  wires:
  Unit Delay/1 -> On_Dly/1
  On/1 -> Unit Delay/1
  Unit Delay1/1 -> Off_Dly/1
  Off/1 -> Unit Delay1/1

== system comparePWM/PWM Gates Generator/Averaging/Delay/NoDelay ==
  On : Inport
  Off : Inport  Port=2
  On_Dly : Outport
  Off_Dly : Outport  Port=2
  wires:
  Off/1 -> Off_Dly/1
  On/1 -> On_Dly/1

== system comparePWM/PWM Gates Generator/Carrier Frequency PWM Generator/Delay/Delay ==
  On : Inport
  Off : Inport  Port=2
  Unit Delay : UnitDelay  SampleTime=1/fsw  HasFrameUpgradeWarning=on
  Unit Delay1 : UnitDelay  SampleTime=1/fsw  HasFrameUpgradeWarning=on
  On_Dly : Outport
  Off_Dly : Outport  Port=2
  wires:
  Unit Delay/1 -> On_Dly/1
  On/1 -> Unit Delay/1
  Unit Delay1/1 -> Off_Dly/1
  Off/1 -> Unit Delay1/1

== system comparePWM/PWM Gates Generator/Carrier Frequency PWM Generator/Delay/NoDelay ==
  On : Inport
  Off : Inport  Port=2
  On_Dly : Outport
  Off_Dly : Outport  Port=2
  wires:
  Off/1 -> Off_Dly/1
  On/1 -> On_Dly/1

== system comparePWM/PWM Gates Generator/Carrier Frequency PWM Generator HL Dead Time/Delay/Delay ==
  On : Inport
  Off : Inport  Port=2
  Unit Delay : UnitDelay  SampleTime=1/fsw  HasFrameUpgradeWarning=on
  Unit Delay1 : UnitDelay  SampleTime=1/fsw  HasFrameUpgradeWarning=on
  On_Dly : Outport
  Off_Dly : Outport  Port=2
  wires:
  Unit Delay/1 -> On_Dly/1
  On/1 -> Unit Delay/1
  Unit Delay1/1 -> Off_Dly/1
  Off/1 -> Unit Delay1/1

== system comparePWM/PWM Gates Generator/Carrier Frequency PWM Generator HL Dead Time/Delay/NoDelay ==
  On : Inport
  Off : Inport  Port=2
  On_Dly : Outport
  Off_Dly : Outport  Port=2
  wires:
  Off/1 -> Off_Dly/1
  On/1 -> On_Dly/1

== system comparePWM/PWM Gates Generator/Fast Simulink PWM Generator/Delay/Delay ==
  On : Inport
  Off : Inport  Port=2
  Unit Delay : UnitDelay  SampleTime=1/fsw  HasFrameUpgradeWarning=on
  Unit Delay1 : UnitDelay  SampleTime=1/fsw  HasFrameUpgradeWarning=on
  On_Dly : Outport
  Off_Dly : Outport  Port=2
  wires:
  Unit Delay/1 -> On_Dly/1
  On/1 -> Unit Delay/1
  Unit Delay1/1 -> Off_Dly/1
  Off/1 -> Unit Delay1/1

== system comparePWM/PWM Gates Generator/Fast Simulink PWM Generator/Delay/NoDelay ==
  On : Inport
  Off : Inport  Port=2
  On_Dly : Outport
  Off_Dly : Outport  Port=2
  wires:
  Off/1 -> Off_Dly/1
  On/1 -> On_Dly/1

== system comparePWM/PWM Gates Generator/Fast Simulink PWM Generator HL Dead Time/Delay/Delay ==
  On : Inport
  Off : Inport  Port=2
  Unit Delay : UnitDelay  SampleTime=1/fsw  HasFrameUpgradeWarning=on
  Unit Delay1 : UnitDelay  SampleTime=1/fsw  HasFrameUpgradeWarning=on
  On_Dly : Outport
  Off_Dly : Outport  Port=2
  wires:
  Unit Delay/1 -> On_Dly/1
  On/1 -> Unit Delay/1
  Unit Delay1/1 -> Off_Dly/1
  Off/1 -> Unit Delay1/1

== system comparePWM/PWM Gates Generator/Fast Simulink PWM Generator HL Dead Time/Delay/NoDelay ==
  On : Inport
  Off : Inport  Port=2
  On_Dly : Outport
  Off_Dly : Outport  Port=2
  wires:
  Off/1 -> Off_Dly/1
  On/1 -> On_Dly/1

== system comparePWM/PWM Gates Generator/Subcycle Averaging/Delay/Delay ==
  On : Inport
  Off : Inport  Port=2
  Unit Delay : UnitDelay  SampleTime=1/fsw  HasFrameUpgradeWarning=on
  Unit Delay1 : UnitDelay  SampleTime=1/fsw  HasFrameUpgradeWarning=on
  On_Dly : Outport
  Off_Dly : Outport  Port=2
  wires:
  Unit Delay/1 -> On_Dly/1
  On/1 -> Unit Delay/1
  Unit Delay1/1 -> Off_Dly/1
  Off/1 -> Unit Delay1/1

== system comparePWM/PWM Gates Generator/Subcycle Averaging/Delay/NoDelay ==
  On : Inport
  Off : Inport  Port=2
  On_Dly : Outport
  Off_Dly : Outport  Port=2
  wires:
  Off/1 -> Off_Dly/1
  On/1 -> On_Dly/1

== matlab function comparePWM/PWM Gates Generator/Averaging/Averaging/Calculate Average Duty Cycles ==
  data: TgabcON input; DC output size=[6,1]; TgabcOFF input; fsw parameter
function DC = fcn(TgabcON,TgabcOFF,fsw)

% Calculate length of subcycle 
Tsw = 1/fsw;
% define size of DC
DC = zeros(6,1);

for p=1:3   % all 3 phases
       DC(p*2-1,1) = (TgabcOFF(p) - TgabcON(p))/Tsw;    
       DC(p*2,1) = 1-  DC(p*2-1,1);
end

== matlab function comparePWM/PWM Gates Generator/Subcycle Averaging/SubcycleAveraging/Calculate Subcycle Duty Cycles ==
  data: TgabcON input; DCss output size=[20,3]; TgabcOFF input; fsw parameter; N parameter
function DCss = fcn(TgabcON,TgabcOFF,fsw,N)

% Calculate length of subcycle 
Tss = 1/fsw/N;
% define size of DCss
DCss = zeros(20,3);

for p=1:3   % all 3 phases
    % Set flag for switching on detection
    Flag = 0;
    
    for i=1:N  % all N subcycle intervals
       switch Flag
           case 0 % till switching on
                if TgabcON(p) < i*Tss
                     if TgabcOFF(p) < i*Tss
                         DCss(i,p) = (TgabcOFF(p) - TgabcON(p))/Tss;
                         Flag = 2;
                     else
                         DCss(i,p) = i - TgabcON(p)/Tss;
                         Flag = 1;
                     end
                else
                    DCss(i,p) = 0;
                end
    
           case 1 % till switching off
                if TgabcOFF(p) < i*Tss
                    DCss(i,p) = TgabcOFF(p)/Tss - (i-1);
                    Flag = 2;
                else
                    DCss(i,p) = 1;
                end

           otherwise % end of cycle
                 DCss(i,p) = 0;
        end
    end
end

== matlab function comparePWM/PWM Gates Generator/Subcycle Averaging/SubcycleAveraging/Output Subcycles ==
  data: DCss input size=[20,3]; DC output size=6; i input
function DC = fcn(DCss, i)

DC = zeros(6,1);

% Output DC per phase
DC = [DCss(i,1); ...
          1-DCss(i,1); ...
          DCss(i,2); ...
          1-DCss(i,2); ...
          DCss(i,3); ...
          1-DCss(i,3)];
